simulink model "solution1_7009"  (R2017b)
settings: Solver=FixedStepAuto  StartTime=0.0  StopTime=inf  FixedStep=0.01  RelTol=1e-3
values from neighbouring files (symbols this model uses):
  g = 9.81    [initialize_simplemodel.m]    (also in initialize_simplemodel_Trial.m; tire_friction_circle.m)
  h = 0.35    [initialize_simplemodel.m]    (also in initialize_simplemodel_Trial.m)
  lf = 1.4    [initialize_simplemodel.m]    (also in initialize_simplemodel_Trial.m)
  lr = 1.345    [initialize_simplemodel.m]    (also in initialize_simplemodel_Trial.m)
  m = 1400    [initialize_simplemodel.m]    (also in initialize_simplemodel_Trial.m = 1300; tire_friction_circle.m = 1300)
  r = 0.34    [initialize_simplemodel.m]    (also in initialize_simplemodel_Trial.m)
  tr = 1.684/2    (= 0.842)    [initialize_simplemodel.m]    (also in initialize_simplemodel_Trial.m)
  v_init = 60*5/18    (= 16.6666666667)    [initialize_simplemodel.m]    (also in initialize_simplemodel_Trial.m)
undefined symbols (not defined in the file or in its folder): DiscIntNeverNeededParam
libraries: simulink x26
(part 2 of 2)

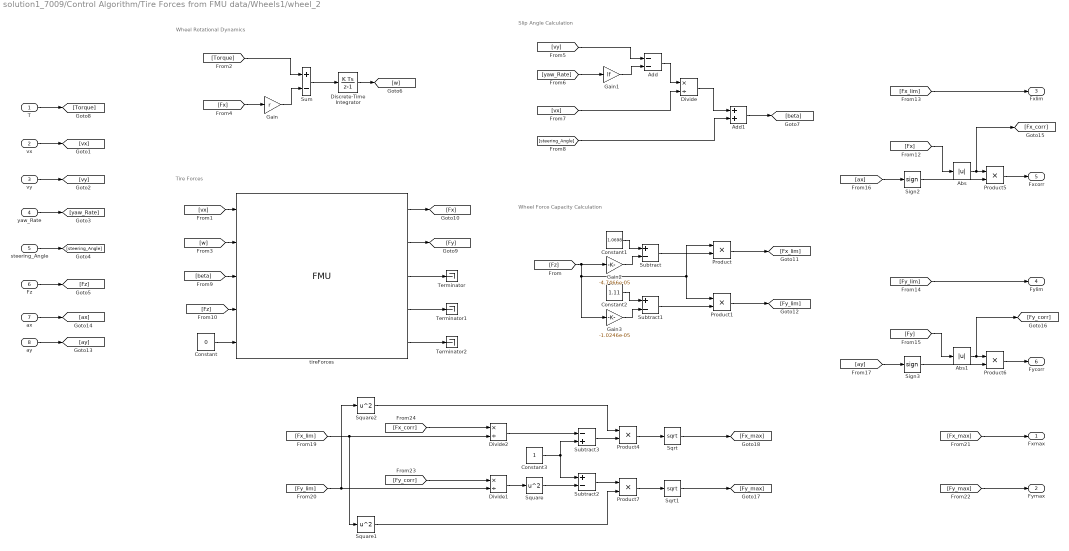
== system solution1_7009/Control Algorithm/Tire Forces from FMU data/Wheels1/wheel_2 ==
  note: Tire Forces
  note: Wheel Rotational Dynamics
  note: Slip Angle Calculation
  note: Wheel Force Capacity Calculation
  T : Inport
  vx : Inport  Port=2
  vy : Inport  Port=3
  yaw_Rate : Inport  Port=4
  steering_Angle : Inport  Port=5
  Fz : Inport  Port=6
  ax : Inport  Port=7
  ay : Inport  Port=8
  Abs : Abs
  Abs1 : Abs
  Add : Sum  Inputs=--
  Add1 : Sum
  Constant : Constant  Value=0
  Constant1 : Constant  Value=1.0698
  Constant2 : Constant  Value=1.11
  Constant3 : Constant
  Discrete-Time Integrator : DiscreteIntegrator  InitialConditionSetting=State (most efficient)  SampleTime=-1  ICPrevOutput=DiscIntNeverNeededParam  ICPrevScaledInput=DiscIntNeverNeededParam
  Divide : Product  Inputs=*/
  Divide1 : Product  Inputs=*/
  Divide2 : Product  Inputs=*/
  Gain : Gain  Gain=r
  Gain1 : Gain  Gain=lf
  Gain2 : Gain  Gain=-4.7466e-05
  Gain3 : Gain  Gain=-1.0246e-05
  Product{,1,4..7} (6 alike) : Product
  Sign2 : Signum
  Sign3 : Signum
  Sqrt : Sqrt  SaturateOnIntegerOverflow=on
  Sqrt1 : Sqrt  SaturateOnIntegerOverflow=on
  Square : Math  Operator=square  RndMeth=Zero  SaturateOnIntegerOverflow=on
  Square1 : Math  Operator=square  RndMeth=Zero  SaturateOnIntegerOverflow=on
  Square2 : Math  Operator=square  RndMeth=Zero  SaturateOnIntegerOverflow=on
  Subtract : Sum  Inputs=+-
  Subtract1 : Sum  Inputs=+-
  Subtract2 : Sum  Inputs=+-
  Subtract3 : Sum  Inputs=-+
  Sum : Sum  Inputs=+-
  Terminator : Terminator
  Terminator1 : Terminator
  Terminator2 : Terminator
  tireForces : FMU  FMUName=MED2018_TireModel.fmu  FMUMode=CoSimulation  FMUSampleTime=-1  mask(TyreFMUContainer [Co-Simulation, v2.0]){}
      mask Display:
      | disp('TyreFMUContainer');
      | port_label('output',1,'Fx');
      | port_label('output',2,'Fy');
      | port_label('output',3,'Mz');
      | port_label('output',4,'r');
      | port_label('output',5,'Mx');
      | port_label('input',1,'vx');
      | port_label('input',2,'w');
      | port_label('input',3,'beta');
      | port_label('input',4,'Fz');
      | port_label('input',5,'camber');
  Fxmax : Outport
  Fymax : Outport  Port=2
  Fxlim : Outport  Port=3
  Fylim : Outport  Port=4
  Fxcorr : Outport  Port=5
  Fycorr : Outport  Port=6
  wires:
  Discrete-Time Integrator/1 -> [w]
  tireForces/5 -> Terminator2/1
  tireForces/2 -> [Fy]
  tireForces/4 -> Terminator1/1
  tireForces/3 -> Terminator/1
  Sum/1 -> Discrete-Time Integrator/1
  [Torque] -> Sum/1
  Gain/1 -> Sum/2
  [Fx] -> Gain/1
  Constant/1 -> tireForces/5
  Gain1/1 -> Add/2
  Add/1 -> Divide/1
  [w] -> tireForces/2
  vx/1 -> [vx]
  vy/1 -> [vy]
  steering_Angle/1 -> [steering_Angle]
  yaw_Rate/1 -> [yaw_Rate]
  Fz/1 -> [Fz]
  [vx] -> tireForces/1
  [vy] -> Add/1
  [yaw_Rate] -> Gain1/1
  [vx] -> Divide/2
  Divide/1 -> Add1/1
  [steering_Angle] -> Add1/2
  Add1/1 -> [beta]
  [beta] -> tireForces/3
  [Fz] -> tireForces/4
  T/1 -> [Torque]
  tireForces/1 -> [Fx]
  Product/1 -> [Fx_lim]
  Product1/1 -> [Fy_lim]
  Subtract1/1 -> Product1/2
  [Fz] -> Gain3/1, Product/1, Product1/1, Gain2/1
  Gain2/1 -> Subtract/2
  Constant1/1 -> Subtract/1
  Gain3/1 -> Subtract1/2
  Constant2/1 -> Subtract1/1
  Subtract/1 -> Product/2
  ay/1 -> [ay]
  ax/1 -> [ax]
  [Fy_max] -> Fymax/1
  [Fx_corr] -> Divide2/1
  Product5/1 -> Fxcorr/1
  Product6/1 -> Fycorr/1
  Abs/1 -> [Fx_corr], Product5/1
  Divide2/1 -> Subtract3/1
  [Fy] -> Abs1/1
  Sign3/1 -> Product6/2
  Divide1/1 -> Square/1
  Product4/1 -> Sqrt/1
  Subtract2/1 -> Product7/1
  Product7/1 -> Sqrt1/1
  Constant3/1 -> Subtract3/2, Subtract2/1
  Abs1/1 -> [Fy_corr], Product6/1
  Square2/1 -> Product4/1
  [Fx_lim] -> Fxlim/1
  [Fy_lim] -> Fylim/1
  [Fy_lim] -> Divide1/2, Square2/1
  Subtract3/1 -> Product4/2
  Sign2/1 -> Product5/2
  Square/1 -> Subtract2/2
  [ay] -> Sign3/1
  [Fx_lim] -> Divide2/2, Square1/1
  [Fx] -> Abs/1
  Sqrt/1 -> [Fx_max]
  [Fx_max] -> Fxmax/1
  [Fy_corr] -> Divide1/1
  [ax] -> Sign2/1
  Sqrt1/1 -> [Fy_max]
  Square1/1 -> Product7/2

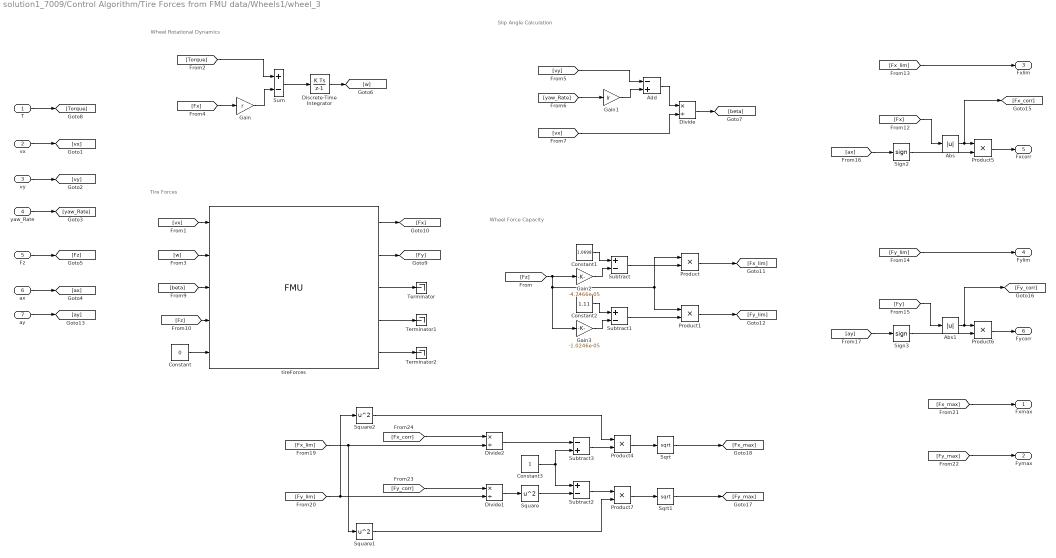
== system solution1_7009/Control Algorithm/Tire Forces from FMU data/Wheels1/wheel_3 ==
  note: Tire Forces
  note: Wheel Rotational Dynamics
  note: Slip Angle Calculation
  note: Wheel Force Capacity
  T : Inport
  vx : Inport  Port=2
  vy : Inport  Port=3
  yaw_Rate : Inport  Port=4
  Fz : Inport  Port=5
  ax : Inport  Port=6
  ay : Inport  Port=7
  Abs : Abs
  Abs1 : Abs
  Add : Sum  Inputs=-+
  Constant : Constant  Value=0
  Constant1 : Constant  Value=1.0698
  Constant2 : Constant  Value=1.11
  Constant3 : Constant
  Discrete-Time Integrator : DiscreteIntegrator  InitialConditionSetting=State (most efficient)  SampleTime=-1  ICPrevOutput=DiscIntNeverNeededParam  ICPrevScaledInput=DiscIntNeverNeededParam
  Divide : Product  Inputs=*/
  Divide1 : Product  Inputs=*/
  Divide2 : Product  Inputs=*/
  Gain : Gain  Gain=r
  Gain1 : Gain  Gain=lr
  Gain2 : Gain  Gain=-4.7466e-05
  Gain3 : Gain  Gain=-1.0246e-05
  Product{,1,4..7} (6 alike) : Product
  Sign2 : Signum
  Sign3 : Signum
  Sqrt : Sqrt  SaturateOnIntegerOverflow=on
  Sqrt1 : Sqrt  SaturateOnIntegerOverflow=on
  Square : Math  Operator=square  RndMeth=Zero  SaturateOnIntegerOverflow=on
  Square1 : Math  Operator=square  RndMeth=Zero  SaturateOnIntegerOverflow=on
  Square2 : Math  Operator=square  RndMeth=Zero  SaturateOnIntegerOverflow=on
  Subtract : Sum  Inputs=+-
  Subtract1 : Sum  Inputs=+-
  Subtract2 : Sum  Inputs=+-
  Subtract3 : Sum  Inputs=-+
  Sum : Sum  Inputs=+-
  Terminator : Terminator
  Terminator1 : Terminator
  Terminator2 : Terminator
  tireForces : FMU  FMUName=MED2018_TireModel.fmu  FMUMode=CoSimulation  FMUSampleTime=-1  mask(TyreFMUContainer [Co-Simulation, v2.0]){}
      mask Display:
      | disp('TyreFMUContainer');
      | port_label('output',1,'Fx');
      | port_label('output',2,'Fy');
      | port_label('output',3,'Mz');
      | port_label('output',4,'r');
      | port_label('output',5,'Mx');
      | port_label('input',1,'vx');
      | port_label('input',2,'w');
      | port_label('input',3,'beta');
      | port_label('input',4,'Fz');
      | port_label('input',5,'camber');
  Fxmax : Outport
  Fymax : Outport  Port=2
  Fxlim : Outport  Port=3
  Fylim : Outport  Port=4
  Fxcorr : Outport  Port=5
  Fycorr : Outport  Port=6
  wires:
  Discrete-Time Integrator/1 -> [w]
  tireForces/5 -> Terminator2/1
  tireForces/2 -> [Fy]
  tireForces/4 -> Terminator1/1
  tireForces/3 -> Terminator/1
  Sum/1 -> Discrete-Time Integrator/1
  [Torque] -> Sum/1
  Gain/1 -> Sum/2
  [Fx] -> Gain/1
  Constant/1 -> tireForces/5
  Gain1/1 -> Add/2
  Add/1 -> Divide/1
  [w] -> tireForces/2
  vx/1 -> [vx]
  vy/1 -> [vy]
  yaw_Rate/1 -> [yaw_Rate]
  Fz/1 -> [Fz]
  [vx] -> tireForces/1
  [vy] -> Add/1
  [yaw_Rate] -> Gain1/1
  [vx] -> Divide/2
  [beta] -> tireForces/3
  [Fz] -> tireForces/4
  T/1 -> [Torque]
  tireForces/1 -> [Fx]
  Divide/1 -> [beta]
  Product/1 -> [Fx_lim]
  Product1/1 -> [Fy_lim]
  Subtract1/1 -> Product1/2
  [Fz] -> Gain3/1, Product/1, Product1/1, Gain2/1
  Gain2/1 -> Subtract/2
  Constant1/1 -> Subtract/1
  Gain3/1 -> Subtract1/2
  Constant2/1 -> Subtract1/1
  Subtract/1 -> Product/2
  ay/1 -> [ay]
  ax/1 -> [ax]
  [Fy_max] -> Fymax/1
  [Fx_corr] -> Divide2/1
  Product5/1 -> Fxcorr/1
  Product6/1 -> Fycorr/1
  Abs/1 -> [Fx_corr], Product5/1
  Divide2/1 -> Subtract3/1
  [Fy] -> Abs1/1
  Sign3/1 -> Product6/2
  Divide1/1 -> Square/1
  Product4/1 -> Sqrt/1
  Subtract2/1 -> Product7/1
  Product7/1 -> Sqrt1/1
  Constant3/1 -> Subtract3/2, Subtract2/1
  Abs1/1 -> [Fy_corr], Product6/1
  Square2/1 -> Product4/1
  [Fx_lim] -> Fxlim/1
  [Fy_lim] -> Fylim/1
  [Fy_lim] -> Divide1/2, Square2/1
  Subtract3/1 -> Product4/2
  Sign2/1 -> Product5/2
  Square/1 -> Subtract2/2
  [ay] -> Sign3/1
  [Fx_lim] -> Divide2/2, Square1/1
  [Fx] -> Abs/1
  Sqrt/1 -> [Fx_max]
  [Fx_max] -> Fxmax/1
  [Fy_corr] -> Divide1/1
  [ax] -> Sign2/1
  Sqrt1/1 -> [Fy_max]
  Square1/1 -> Product7/2

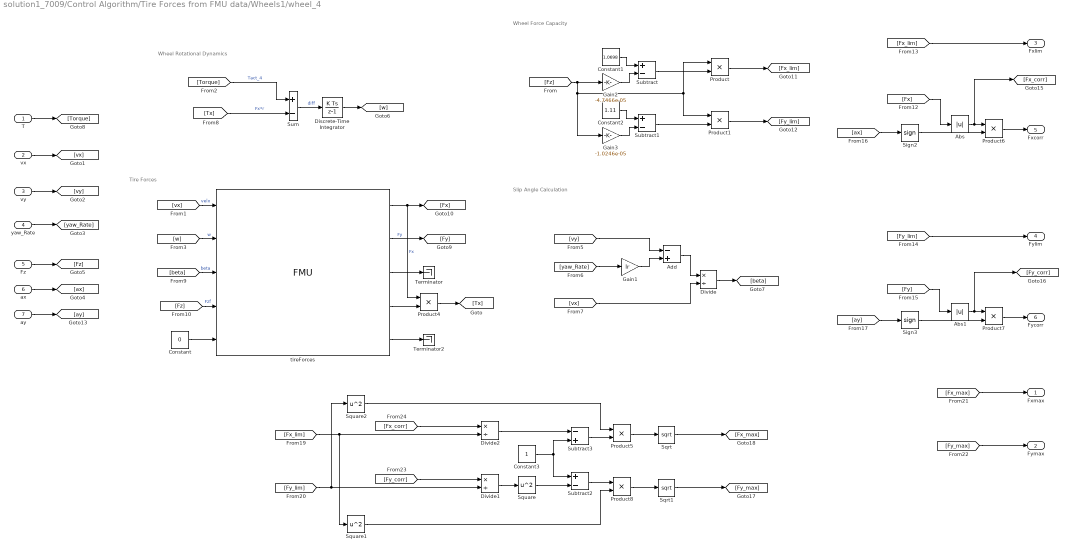
== system solution1_7009/Control Algorithm/Tire Forces from FMU data/Wheels1/wheel_4 ==
  note: Tire Forces
  note: Wheel Rotational Dynamics
  note: Slip Angle Calculation
  note: Wheel Force Capacity
  T : Inport
  vx : Inport  Port=2
  vy : Inport  Port=3
  yaw_Rate : Inport  Port=4
  Fz : Inport  Port=5
  ax : Inport  Port=6
  ay : Inport  Port=7
  Abs : Abs
  Abs1 : Abs
  Add : Sum  Inputs=-+
  Constant : Constant  Value=0
  Constant1 : Constant  Value=1.0698
  Constant2 : Constant  Value=1.11
  Constant3 : Constant
  Discrete-Time Integrator : DiscreteIntegrator  InitialCondition=v_init/r  InitialConditionSetting=State (most efficient)  SampleTime=-1  ICPrevOutput=DiscIntNeverNeededParam  ICPrevScaledInput=DiscIntNeverNeededParam
  Divide : Product  Inputs=*/
  Divide1 : Product  Inputs=*/
  Divide2 : Product  Inputs=*/
  Gain1 : Gain  Gain=lr
  Gain2 : Gain  Gain=-4.7466e-05
  Gain3 : Gain  Gain=-1.0246e-05
  Product{,1,4..8} (7 alike) : Product
  Sign2 : Signum
  Sign3 : Signum
  Sqrt : Sqrt  SaturateOnIntegerOverflow=on
  Sqrt1 : Sqrt  SaturateOnIntegerOverflow=on
  Square : Math  Operator=square  RndMeth=Zero  SaturateOnIntegerOverflow=on
  Square1 : Math  Operator=square  RndMeth=Zero  SaturateOnIntegerOverflow=on
  Square2 : Math  Operator=square  RndMeth=Zero  SaturateOnIntegerOverflow=on
  Subtract : Sum  Inputs=+-
  Subtract1 : Sum  Inputs=+-
  Subtract2 : Sum  Inputs=+-
  Subtract3 : Sum  Inputs=-+
  Sum : Sum  Inputs=+-
  Terminator : Terminator
  Terminator2 : Terminator
  tireForces : FMU  FMUName=MED2018_TireModel.fmu  FMUDebugLogging=on  FMUMode=CoSimulation  FMUSampleTime=-1  mask(TyreFMUContainer [Co-Simulation, v2.0]){}
      mask Display:
      | disp('TyreFMUContainer');
      | port_label('output',1,'Fx');
      | port_label('output',2,'Fy');
      | port_label('output',3,'Mz');
      | port_label('output',4,'r');
      | port_label('output',5,'Mx');
      | port_label('input',1,'vx');
      | port_label('input',2,'w');
      | port_label('input',3,'beta');
      | port_label('input',4,'Fz');
      | port_label('input',5,'camber');
  Fxmax : Outport
  Fymax : Outport  Port=2
  Fxlim : Outport  Port=3
  Fylim : Outport  Port=4
  Fxcorr : Outport  Port=5
  Fycorr : Outport  Port=6
  wires:
  Discrete-Time Integrator/1 -> [w]
  tireForces/5 -> Terminator2/1
  tireForces/2 -> [Fy]  "Fy"
  tireForces/4 -> Product4/2
  tireForces/3 -> Terminator/1
  Sum/1 -> Discrete-Time Integrator/1  "diff"
  [Torque] -> Sum/1  "Tact_4"
  [Tx] -> Sum/2  "Fx*r"
  Constant/1 -> tireForces/5
  [w] -> tireForces/2  "w"
  vx/1 -> [vx]
  vy/1 -> [vy]
  yaw_Rate/1 -> [yaw_Rate]
  Fz/1 -> [Fz]
  [vx] -> tireForces/1  "velx"
  [beta] -> tireForces/3  "beta"
  [Fz] -> tireForces/4  "Fzf"
  T/1 -> [Torque]
  tireForces/1 -> Product4/1, [Fx]  "Fx"
  [vy] -> Add/1
  [vx] -> Divide/2
  [yaw_Rate] -> Gain1/1
  Add/1 -> Divide/1
  Gain1/1 -> Add/2
  Divide/1 -> [beta]
  Product/1 -> [Fx_lim]
  Product1/1 -> [Fy_lim]
  Subtract1/1 -> Product1/2
  [Fz] -> Gain3/1, Product/1, Product1/1, Gain2/1
  Gain2/1 -> Subtract/2
  Constant1/1 -> Subtract/1
  Gain3/1 -> Subtract1/2
  Constant2/1 -> Subtract1/1
  Subtract/1 -> Product/2
  Product4/1 -> [Tx]
  ay/1 -> [ay]
  ax/1 -> [ax]
  Divide1/1 -> Square/1
  Sign3/1 -> Product7/2
  [Fy_max] -> Fymax/1
  Product7/1 -> Fycorr/1
  Abs/1 -> [Fx_corr], Product6/1
  Sqrt1/1 -> [Fy_max]
  Square1/1 -> Product8/2
  Sqrt/1 -> [Fx_max]
  [Fx_max] -> Fxmax/1
  [ay] -> Sign3/1
  [Fx] -> Abs/1
  Square/1 -> Subtract2/2
  Subtract3/1 -> Product5/2
  Product6/1 -> Fxcorr/1
  [Fx_lim] -> Fxlim/1
  Square2/1 -> Product5/1
  [Fx_corr] -> Divide2/1
  [ax] -> Sign2/1
  [Fx_lim] -> Divide2/2, Square1/1
  [Fy] -> Abs1/1
  [Fy_lim] -> Divide1/2, Square2/1
  Sign2/1 -> Product6/2
  [Fy_lim] -> Fylim/1
  Subtract2/1 -> Product8/1
  Abs1/1 -> [Fy_corr], Product7/1
  Product5/1 -> Sqrt/1
  Divide2/1 -> Subtract3/1
  [Fy_corr] -> Divide1/1
  Constant3/1 -> Subtract3/2, Subtract2/1
  Product8/1 -> Sqrt1/1

== system solution1_7009/Control Algorithm/Control/Drift generate/Max wheel force/Wheel Traction control ==
  Txmargin : Inport
  Abs : Abs
  Abs1 : Abs
  Demux : Demux
  Max : MinMax  Inputs=2
  cmd_Tx_3 : Outport
  "cmd_Tx_4 " : Outport  Port=2
  wires:
  Abs/1 -> Max/1
  [Tmax_3] -> Abs/1  "Tx3_max"
  Demux/4 -> [Tmax_4]
  Demux/3 -> [Tmax_3]
  Demux/2 -> [Tmax_2]
  Demux/1 -> [Tmax_1]
  Txmargin/1 -> Demux/1
  [Tmax_4] -> Abs1/1  "Tx4_max"
  Abs1/1 -> Max/2
  Max/1 -> cmd_Tx_3/1, "cmd_Tx_4 "/1

== matlab function solution1_7009/Control Algorithm/Tire Forces from FMU data/Tire Vertical Load ==
  data: ax input; ay input; Fz output; g parameter; h parameter; lf parameter; lr parameter; m parameter; tf parameter; tr parameter
function Fz  = vehicleModel(ax, ay, g, h, lf, lr, m, tf, tr)

% Function to calculate vertical loads
% Vehicle Parameters must be loaded from init.m

%Load Equations

Fz = [m*g*lr/(lf+lr)/2;m*g*lr/(lf+lr)/2;m*g*lf/(lf+lr)/2;m*g*lf/(lf+lr)/2];
Fz(1) = m * (g*lr/(lf+lr)/2 - ax*h/(lf+lr)/2 - ay*h/tf/2);
Fz(2) = m * (g*lr/(lf+lr)/2 - ax*h/(lf+lr)/2 + ay*h/tf/2);
Fz(3) = m * (g*lf/(lf+lr)/2 + ax*h/(lf+lr)/2 - ay*h/tr/2);
Fz(4) = m * (g*lf/(lf+lr)/2 + ax*h/(lf+lr)/2 + ay*h/tr/2);
